simulink model "Oving3Oppg2c"  (R2020b)
settings: Solver=VariableStepAuto  StartTime=0.0  StopTime=100  MaxStep=0.01  RelTol=1e-3
settings Model: Creator=crezl  LastModifiedBy=crezl

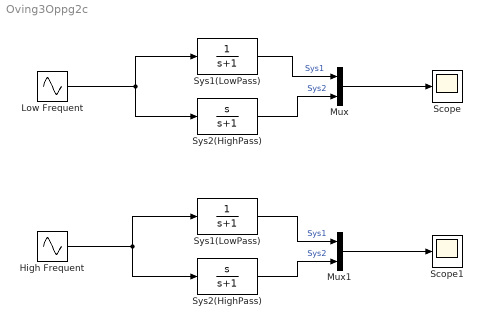
== system Oving3Oppg2c ==
  High Frequent : Sin  Frequency=10  SampleTime=0
  Low Frequent : Sin  Frequency=0.1  SampleTime=0
  Mux : Mux  Inputs=2
  Mux1 : Mux  Inputs=2
  Scope : Scope
  Scope1 : Scope
  Sys1(LowPass) : TransferFcn  Denominator=[1 1]
  "Sys1(LowPass) " : TransferFcn  Denominator=[1 1]
  Sys2(HighPass) : TransferFcn  Numerator=[1 0]  Denominator=[1 1]
  "Sys2(HighPass) " : TransferFcn  Numerator=[1 0]  Denominator=[1 1]
  wires:
  Low Frequent/1 -> Sys1(LowPass)/1, Sys2(HighPass)/1
  High Frequent/1 -> "Sys2(HighPass) "/1, "Sys1(LowPass) "/1
  "Sys2(HighPass) "/1 -> Mux1/2  "Sys2"
  "Sys1(LowPass) "/1 -> Mux1/1  "Sys1"
  Sys2(HighPass)/1 -> Mux/2  "Sys2"
  Sys1(LowPass)/1 -> Mux/1  "Sys1"
  Mux/1 -> Scope/1
  Mux1/1 -> Scope1/1
